simulink model "IntelligentBinPicking"  (R2024a)
settings: Solver=FixedStepAuto  StartTime=0.0  StopTime=200  FixedStep=0.05  RelTol=1e-3
PreLoadFcn:
  | initRobotModelParam;
model workspace (MAT data in the model file):
  SL_ROS_VariableLengthArrays_MaxSizes : object (value not decoded)
undefined symbols (not defined in the file): binActorRotationSequenceInfo, binActorTranslationSequenceInfo, binCenterPosition, camera_rot, cameraIntrinsics, cx_camera, cy_camera, downSampleForTrajectoryWaypoints, Enable, enumCmd, f, graspRegionTranslation, gray, homePosition, IsAccValid, IsMoving, IsPosValid, isSingleDetection, IsValid, IsVelValid, JointAcc, JointCurrent, JointPos, JointTrajectory, JointVel, maxVisionObjects, Mode, motionPlannerCmdInitValue, motionPlannerResponseInitValue, NumObjects, NumPoints, objectDetectorResponseInitValue, Objects, ObjectTypesID, pickAllOrder, PickAllOrder, PickAndPlaceModes, PickSelectedObjectID, posTargetError, predictionConfidenceScore, RequestID, Reset, RGBCameraTransform, robotCommandInitValue, robotFeedbackInitValue, Sim3dSensor, Status, TargetEETranslation, targetEnv, TaskPlannerSampleTime, Time, TooltipTransform, ur5e
libraries: sim3dlib x13, robotlib x6, robotmaniplib x4, robotcorelib x1, robotsim3dlib x1, sim3dcameralib x1
(part 2 of 2)

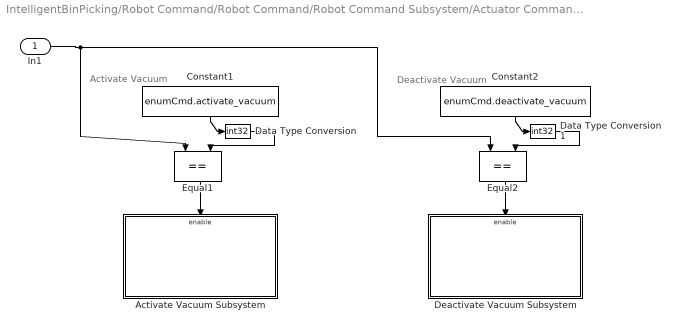
== system IntelligentBinPicking/Robot Command/Robot Command/Robot Command Subsystem/Actuator Commands/Gazebo ==
  note: Deactivate Vacuum
  note: Activate Vacuum
  In1 : Inport
  Activate Vacuum Subsystem : Subsystem
  Constant1 : Constant  Value=enumCmd.activate_vacuum
  Constant2 : Constant  Value=enumCmd.deactivate_vacuum
  Data Type Conversion : DataTypeConversion  OutDataTypeStr=int32  SaturateOnIntegerOverflow=off  RndMeth=Floor
  Data Type Conversion1 : DataTypeConversion  OutDataTypeStr=int32  SaturateOnIntegerOverflow=off  RndMeth=Floor
  Deactivate Vacuum Subsystem : Subsystem
  Equal1 : RelationalOperator  Operator===  OutDataTypeStr=boolean  RndMeth=Simplest  InputSameDT=off
  Equal2 : RelationalOperator  Operator===  OutDataTypeStr=boolean  RndMeth=Simplest  InputSameDT=off
  wires:
  Constant1/1 -> Data Type Conversion/1
  Equal2/1 -> Deactivate Vacuum Subsystem/Enable
  Constant2/1 -> Data Type Conversion1/1
  Equal1/1 -> Activate Vacuum Subsystem/Enable
  In1/1 -> Equal2/1, Equal1/1
  Data Type Conversion/1 -> Equal1/2
  Data Type Conversion1/1 -> Equal2/2

== system IntelligentBinPicking/Robot Command/Robot Command/Robot Command Subsystem/Actuator Commands/Hardware ==
  note: Activate_Deactivate Vacuum
  In1 : Inport
  Activate Vacuum Subsystem : Subsystem
  Constant1 : Constant  Value=enumCmd.activate_vacuum
  Constant2 : Constant  Value=enumCmd.deactivate_vacuum
  Data Type Conversion : DataTypeConversion  OutDataTypeStr=int32  SaturateOnIntegerOverflow=off  RndMeth=Floor
  Data Type Conversion1 : DataTypeConversion  OutDataTypeStr=int32  SaturateOnIntegerOverflow=off  RndMeth=Floor
  Equal1 : RelationalOperator  Operator===  OutDataTypeStr=boolean  RndMeth=Simplest  InputSameDT=off
  Equal2 : RelationalOperator  Operator===  OutDataTypeStr=boolean  RndMeth=Simplest  InputSameDT=off
  OR : Logic  Operator=OR  AllPortsSameDT=off  OutDataTypeStr=boolean
  wires:
  Constant1/1 -> Data Type Conversion1/1
  Equal1/1 -> OR/1
  In1/1 -> Equal1/2, Equal2/1
  Constant2/1 -> Data Type Conversion/1
  Equal2/1 -> OR/2
  OR/1 -> Activate Vacuum Subsystem/Enable
  Data Type Conversion/1 -> Equal2/2
  Data Type Conversion1/1 -> Equal1/1

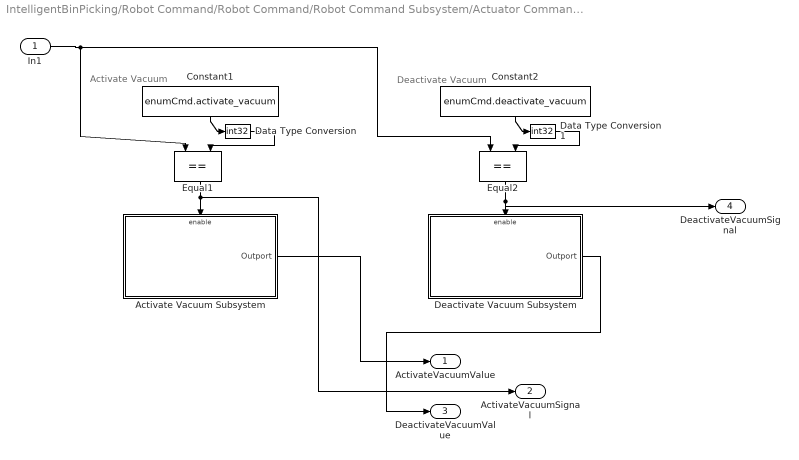
== system IntelligentBinPicking/Robot Command/Robot Command/Robot Command Subsystem/Actuator Commands/Sim3d ==
  note: Deactivate Vacuum
  note: Activate Vacuum
  In1 : Inport
  Activate Vacuum Subsystem : Subsystem
  Constant1 : Constant  Value=enumCmd.activate_vacuum
  Constant2 : Constant  Value=enumCmd.deactivate_vacuum
  Data Type Conversion : DataTypeConversion  OutDataTypeStr=int32  SaturateOnIntegerOverflow=off  RndMeth=Floor
  Data Type Conversion1 : DataTypeConversion  OutDataTypeStr=int32  SaturateOnIntegerOverflow=off  RndMeth=Floor
  Deactivate Vacuum Subsystem : Subsystem
  Equal1 : RelationalOperator  Operator===  OutDataTypeStr=boolean  RndMeth=Simplest  InputSameDT=off
  Equal2 : RelationalOperator  Operator===  OutDataTypeStr=boolean  RndMeth=Simplest  InputSameDT=off
  ActivateVacuumValue : Outport
  ActivateVacuumSignal : Outport  Port=2
  DeactivateVacuumValue : Outport  Port=3
  DeactivateVacuumSignal : Outport  Port=4
  wires:
  Constant1/1 -> Data Type Conversion/1
  Equal2/1 -> DeactivateVacuumSignal/1, Deactivate Vacuum Subsystem/Enable
  Constant2/1 -> Data Type Conversion1/1
  Equal1/1 -> ActivateVacuumSignal/1, Activate Vacuum Subsystem/Enable
  In1/1 -> Equal2/1, Equal1/1
  Data Type Conversion/1 -> Equal1/2
  Data Type Conversion1/1 -> Equal2/2
  Activate Vacuum Subsystem/1(Outport) -> ActivateVacuumValue/1
  Deactivate Vacuum Subsystem/1(Outport) -> DeactivateVacuumValue/1

== system IntelligentBinPicking/Robot Command/Robot Command/Robot Command Subsystem/Actuator Commands/Gazebo/Activate Vacuum Subsystem ==
  Enable : EnablePort
  Activate Vacuum : robotlib/Call Service  topicSource=Select from ROS network  service=/ur5/epick1/on  serviceType=std_srvs/Empty  connectionTimeout=5  keepPersistent=off  ShowErrorCodeOutput=on  legacyBusStruct=off
  Blank Message : robotlib/Blank Message  messageClass=Service Request  entityType=std_srvs/Empty  messageType=std_srvs/EmptyRequest  SampleTime=inf  legacyBusStruct=off
  wires:
  Blank Message/1 -> Activate Vacuum/1

== system IntelligentBinPicking/Robot Command/Robot Command/Robot Command Subsystem/Actuator Commands/Gazebo/Deactivate Vacuum Subsystem ==
  Enable : EnablePort
  Blank Message : robotlib/Blank Message  messageClass=Service Request  entityType=std_srvs/Empty  messageType=std_srvs/EmptyRequest  SampleTime=inf  legacyBusStruct=off
  Deactivate Vacuum : robotlib/Call Service  topicSource=Select from ROS network  service=/ur5/epick1/off  serviceType=std_srvs/Empty  connectionTimeout=5  keepPersistent=off  ShowErrorCodeOutput=on  legacyBusStruct=off
  wires:
  Blank Message/1 -> Deactivate Vacuum/1

== system IntelligentBinPicking/Robot Command/Robot Command/Robot Command Subsystem/Actuator Commands/Hardware/Activate Vacuum Subsystem ==
  Enable : EnablePort
  Activate_Deactivate Vacuum : robotlib/Call Service  topicSource=Specify your own  service=/ur_hardware_interface/hand_back_control  serviceType=std_srvs/Trigger  connectionTimeout=5  keepPersistent=off  ShowErrorCodeOutput=on  legacyBusStruct=off
  Blank Message : robotlib/Blank Message  messageClass=Service Request  entityType=std_srvs/Trigger  messageType=std_srvs/TriggerRequest  SampleTime=inf  legacyBusStruct=off
  wires:
  Blank Message/1 -> Activate_Deactivate Vacuum/1

== system IntelligentBinPicking/Robot Command/Robot Command/Robot Command Subsystem/Actuator Commands/Sim3d/Activate Vacuum Subsystem ==
  Enable : EnablePort
  Constant : Constant  OutDataTypeStr=boolean
  Outport : Outport
  wires:
  Constant/1 -> Outport/1

== system IntelligentBinPicking/Robot Command/Robot Command/Robot Command Subsystem/Actuator Commands/Sim3d/Deactivate Vacuum Subsystem ==
  Enable : EnablePort
  Constant : Constant  Value=0  OutDataTypeStr=boolean
  Outport : Outport
  wires:
  Constant/1 -> Outport/1

== matlab function IntelligentBinPicking/Robot Command/Robot Configuration  Manager/getLastPlannerWaypointConfiguration fcn ==
  data: trajectoryWaypoint input; lastPlannerWaypointConfiguration output size=[1,6]
function lastPlannerWaypointConfiguration = getLastPlannerWaypointConfiguration(trajectoryWaypoint)
lastPlannerWaypointConfiguration=zeros(1,6);
if size(trajectoryWaypoint,2) ==1
    ind=1;
else
    ind=find(all(trajectoryWaypoint == 0), 1, 'first')-1;
end
pose=trajectoryWaypoint(:,ind)';
lastPlannerWaypointConfiguration(1,1:6)=pose;

== matlab function IntelligentBinPicking/Robot Command/Robot Configuration  Manager/getGripperStatus fcn ==
  data: gripperStatus output size=[1,1]; flagG1 input; flagG2 input; graspGT input
function gripperStatus = getGripperStatus(flagG1,flagG2,graspGT)

% Persistent variable to contains state in between fcn call
persistent resultGripper;
persistent flag1GLastStatus;
persistent flag2GLastStatus;
persistent graspGTLastStatus;
if isempty (resultGripper)
    resultGripper =0;
    flag1GLastStatus= false;
    flag2GLastStatus = false;
    graspGTLastStatus =true;
end
if flagG1 || graspGT
    resultGripper= 1;
    flag1GLastStatus = flagG1;
    flag2GLastStatus = false;
    graspGTLastStatus =true;
elseif flag1GLastStatus && ~flagG2
    resultGripper=1; 
end
if flagG1 && flagG2
    resultGripper =1;
end

if ~flagG1 && ~flagG2 && ~flag2GLastStatus && ~flag1GLastStatus
    if graspGTLastStatus
        resultGripper =1;
    else
        resultGripper =0 ;
    end
end

if flagG2 
    resultGripper= 0;
    flag2GLastStatus = flagG2;
    flag1GLastStatus = false;
    graspGTLastStatus =false;
elseif flag2GLastStatus && ~flagG1
    resultGripper=0; 
end

gripperStatus = resultGripper;

== matlab function IntelligentBinPicking/Robot Command/Robot Configuration  Manager/getTrajectoryStatus fcn ==
  data: trajectoryStatus output size=[1,1]; flag1 input; flag2 input
function trajectoryStatus = getTrajectoryStatus(flag1,flag2)

% Persistent variable to contain state in between fcn call
persistent resultTrajectory;
persistent flag1LastStatus;
persistent flag2LastStatus;
if isempty (resultTrajectory)
    resultTrajectory =0;
    flag1LastStatus= false;
    flag2LastStatus = false;
end
if flag1 
    resultTrajectory= 1;
    flag1LastStatus = flag1;
    flag2LastStatus = false;
elseif flag1LastStatus && ~flag2
    resultTrajectory=1; 
end
if flag1 && flag2
    resultTrajectory =1;
end

if ~flag1 && ~flag2 && ~flag2LastStatus && ~flag1LastStatus
    resultTrajectory =0;
end

if flag2 
    resultTrajectory= 0;
    flag2LastStatus = flag2;
    flag1LastStatus = false;
elseif flag2LastStatus && ~flag1
    resultTrajectory=0; 
end

trajectoryStatus = resultTrajectory;

== matlab function IntelligentBinPicking/Object Detector/MATLAB Function ==
  data: objectDetectorResponseIn input Bus: BUS_object_detector_response; objectPose input; objectResponseOut output Bus: BUS_motion_planner_collision_object size=[maxVisionObjects 1]
function objectResponseOut = setObjectDetectedBus(objectDetectorResponseIn,objectPose)

objectResponseOut = objectDetectorResponseIn.Objects;
for i=1:size(objectPose,1)
    objectResponseOut(i).PickPos = objectPose(i, 1:3)';
    objectResponseOut(i).PickEulZYX = [objectPose(i, 4);0;0];
    objectResponseOut(i).ID = ObjectTypesID(objectPose(i, 5));
end

== matlab function IntelligentBinPicking/Robot Command/Robot Configuration  Manager/getRobotConfig fcn ==
  data: trajectoryWaypoint input; robotConfig output size=[6,1]; flag input; homePosition input; subSample input; tasks input
function robotConfig = getRobotConfig(trajectoryWaypoint,flag,homePosition,subSample,tasks)

% Persistent variable to contain state between fcn call
persistent index;
persistent lastTasksStatus;
if isempty (index)
    index=1;   
    trajectoryWaypoint= homePosition;
    lastTasksStatus = ['Place' char(repmat(' ', 1, 251))];
end
type = tasks(1).Type;
type = char(type(type~=0));
if flag 

    if ~strncmp(type,lastTasksStatus,length(type))
        index =1;
    end

    taskStatusPadded = [type char(repmat(' ', 1, 256-length(type)))];
    lastTasksStatus = taskStatusPadded(1:256);

    if strncmp(type, 'Place',5) && size(trajectoryWaypoint,2) ==1
        index =1;
    end
    
end


if ~isempty(trajectoryWaypoint)
    robotConfig = trajectoryWaypoint(1:6,index);
else
    robotConfig = homePosition;
end

if index <=size(trajectoryWaypoint,2)
    index =index + subSample;
    if index >=size(trajectoryWaypoint,2)
        index = size(trajectoryWaypoint,2);
    end
else
    index = size(trajectoryWaypoint,2);
end

== matlab function IntelligentBinPicking/Robot Command/Robot Configuration  Manager/getTargetBinActorName fcn ==
  data: u input; targetBinActorName output string; actorTranslationConfig input; actorRotationConfig input; targetBinActorOrientation output
function [targetBinActorName, targetBinActorOrientation] = getTargetBinActorName(u,actorTranslationConfig,actorRotationConfig)
translation=u(1:3,4)';

minDistance = inf; % Adjust the tolerance as needed
minIndex = 1;
for i = 1:size(actorTranslationConfig, 1)
    % distance = max(abs(givenConfigValues - bins(i, :)'));
    distance = norm(translation(1,1:2) - actorTranslationConfig(i, 1:2)*[1 0 ; 0 -1]);
    if distance < minDistance
        minDistance = distance;
        minIndex = i;
    end
end

if minIndex > 0
    out = string(sprintf('binActor%d', int8(minIndex)));
else
    out = string(sprintf('binActor%d', int8(1)));
end
targetBinActorName=out;
targetBinActorOrientation = [actorRotationConfig(minIndex,1),0,0];

== stateflow chart IntelligentBinPicking/TaskPlanner/Chart ==
  state Setup
    entry:
    ii = 1;
    obsObjectCounter = 1;
    MotionPlannerCmd = motionPlannerCmdInitValue;
    RobotCommand = robotCommandInitValue;
    pickAllObjectIndex = uint32(1);
    objectToPickIndex  = uint32(0);
    objectPickedIndices = zeros(1,maxVisionObjects);
    isVacuumOn = false;
    SimFailed = false;
  state DeactivateVacuum
    entry:
    disp('Sending Deactivate Vacuum Command');
    RobotCommand.CommandToProcess = int32(enumCmd.deactivate_vacuum);
    RobotCommand.ProcessCommand = true;
    exit:
    RobotCommand.ProcessCommand = false;
    isVacuumOn = false;
  state SendToHome
    entry:
    disp('Sending robot to home position');
    RobotCommand.CommandToProcess = int32(enumCmd.send_to_home);
    RobotCommand.ProcessCommand = true;
    exit:
    RobotCommand.ProcessCommand = false;
  state ObjectDetectorFailed
    entry:
    disp(" ");
    disp(" ");
    disp("No objects detected");
    SimFailed = true;
  state DetectObjects
    state SendObjectDetectorRequest
      en: ObjectDetectorRequest;
      disp('Object Detection in Progress');
      %du: ObjectDetectorRequest;
    state ExtractObjectToPickSingleDetection
      en:
      motionCmdWithCollisionObjects = addCollisionObjectsInfo(ObjectDetectorResponse);
      generateDroppingPoses(ObjectDetectorResponse);
      [isObjectInScene, objectToPickPos, objectToPickEul, objectToPickIndex, pickAllObjectIndex] = getObjectToPick(UserCommand, ObjectDetectorResponse, pickAllObjectIndex);
    (junction 417) -> ExtractObjectToPickSingleDetection [order 1] : [isSingleDetection == true && UserCommand.Enable == true && ObjectDetectorResponse.Status == 1 && ...
        | ObjectDetectorResponse.NumObjects >= 1]
    (junction 417) -> SendObjectDetectorRequest [order 2]
    ExtractObjectToPickSingleDetection -> SendObjectDetectorRequest [order 3]
    SendObjectDetectorRequest -> ExtractObjectToPickSingleDetection [order 2] : [UserCommand.Enable == true && ObjectDetectorResponse.Status == 1 && ...
        | ObjectDetectorResponse.NumObjects >= 1]
    ExtractObjectToPickSingleDetection -> (junction 438) [order 2] : [isObjectInScene == true]
  state StopSimulation
    entry:
    objectPickedIndices = zeros(1, maxVisionObjects);
    Stop();
  state GoToPickingPose
    state GetPickingTrajectoryFromMotionPlanner
      entry:
      % Here based on object Pos and Eul get picking pose
      pickPos = objectToPickPos + [0.0; 0.0; 0.01];  % Bring the arm to 1cm above the pick position
      pickEul = objectToPickEul;
      %Create a motion planner task bus
      MotionPlannerCmd = createMotionTask(int32(objectToPickIndex), 'Pick', uint32(300), 0.2, RobotFeedback.JointPos, pickPos, objectToPickEul);
      % Add obstacle objects
      MotionPlannerCmd.NumObstacleObjects = ObjectDetectorResponse.NumObjects - 1;
      ii= 1;
      obsObjectCounter = 1;
      for ii = 1:(ObjectDetectorResponse.NumObjects)
      if objectToPickIndex ~= ii
      MotionPlannerCmd.ObstacleObjects(obsObjectCounter) = ObjectDetectorResponse.Objects(ii);
      obsObjectCounter = obsObjectCounter + 1;
      end
      end
      % Send request to motion planner
      MotionPlannerRequest;
    state SendPickingTrajectoryToRobot
      entry:
      % Send trajectory to driver
      disp("Send traj to robot");
      RobotCommand.JointTrajectory = MotionPlannerResponse.JointTrajectory;
      RobotCommand.CommandToProcess = int32(enumCmd.precomputed_joint_trj);
      RobotCommand.ProcessCommand = true;
      posErr = Inf;
      orErr = Inf;
      success = false;
      during:
      RobotCommand.ProcessCommand = false;
      %  Check error and exit when tooltip reaches desired pose.
      T_task = eul2tform(pickEul');
      T_task(1:3,4) = pickPos;
      if targetEnv == TargetEnvs.Gazebo || targetEnv == TargetEnvs.Sim3d
      [posErr, orErr] = calcTaskSE3MaxError(T_task, RobotFeedback.TooltipTransform);
      if posErr < posTargetError
      success = true;
      end
      else
      success = ~RobotFeedback.IsMoving;
      end
      exit:
    GetPickingTrajectoryFromMotionPlanner -> (junction 14) : [MotionPlannerResponse.RequestID == MotionPlannerCmd.RequestID]
    (junction 14) -> SendPickingTrajectoryToRobot [order 1] : [MotionPlannerResponse.Status == 1 && ...
        | MotionPlannerResponse.IsPosValid == 1 && ...
        | MotionPlannerResponse.IsVelValid == 1 &&...
        |  MotionPlannerResponse.IsAccValid == 1]
  state MotionPlannerFailed
    en:
    disp('Motion Planner failed');
    SimFailed = true;
  state ActivateVacuum
    entry:
    disp('Sending Activate Vacuum Command');
    RobotCommand.CommandToProcess = int32(enumCmd.activate_vacuum);
    RobotCommand.ProcessCommand = true;
    exit:
    RobotCommand.ProcessCommand = false;
    isVacuumOn = true;
  state GoToDroppingPose
    state RequestDroppingTrajectoryFromMotionPlanner
      entry:
      droppingPose = getDroppingPose(ObjectDetectorResponse,objectToPickIndex,droppingPoses, RobotFeedback.TooltipTransform);
      % Create motion planner task bus
      MotionPlannerCmd = createMotionTask(int32(objectToPickIndex), 'Place', uint32(300), 0.2, RobotFeedback.JointPos, droppingPose(1:3), droppingPose(4:6));
      % Add obstacle objects
      MotionPlannerCmd.NumObstacleObjects = ObjectDetectorResponse.NumObjects - 1;
      ii= 1;
      obsObjectCounter = 1;
      for ii = 1:(ObjectDetectorResponse.NumObjects)
      if objectToPickIndex ~= ii
      MotionPlannerCmd.ObstacleObjects(obsObjectCounter) = ObjectDetectorResponse.Objects(ii);
      obsObjectCounter = obsObjectCounter + 1;
      end
      end
      % Send request to motion planner
      MotionPlannerRequest;
    state SendDroppingTrajectoryToRobot
      entry:
      % Send trajectory to driver
      RobotCommand.JointTrajectory = MotionPlannerResponse.JointTrajectory;
      RobotCommand.CommandToProcess = int32(enumCmd.precomputed_joint_trj);
      RobotCommand.ProcessCommand = true;
      posErr = Inf;
      orErr = Inf;
      success = false;
      during:
      RobotCommand.ProcessCommand = false;
      %  Check error and exit when tooltip reaches desired pose.
      T_task = eul2tform(droppingPose(4:6)');
      T_task(1:3,4) = droppingPose(1:3);
      if targetEnv == TargetEnvs.Gazebo || targetEnv == TargetEnvs.Sim3d
      [posErr, orErr] = calcTaskSE3MaxError(T_task, RobotFeedback.TooltipTransform);
      if posErr < posTargetError
      success = true;
      end
      else
      success = ~RobotFeedback.IsMoving;
      end
      exit:
    RequestDroppingTrajectoryFromMotionPlanner -> (junction 128) : [MotionPlannerResponse.RequestID == MotionPlannerCmd.RequestID]
    (junction 128) -> SendDroppingTrajectoryToRobot [order 1] : [MotionPlannerResponse.Status == 1 && ...
        | MotionPlannerResponse.IsPosValid == 1 && ...
        | MotionPlannerResponse.IsVelValid == 1 && ...
        | MotionPlannerResponse.IsAccValid == 1]
  state Stop [function]
  SendPickingTrajectoryToRobot -> ActivateVacuum : [success == true]
  SendToHome -> (junction 417) [order 2]
  ActivateVacuum -> RequestDroppingTrajectoryFromMotionPlanner : {pause(0.5)}
  ExtractObjectToPickSingleDetection -> StopSimulation [order 1] : [objectToPickIndex == uint32(-1)]
      | {disp('No more objects to pick. Stopping simulation')}
  (junction 438) -> GetPickingTrajectoryFromMotionPlanner : {pause(1)}
  (default) -> Setup
  Setup -> (junction 498) : [UserCommand.Enable == true && RobotFeedback.IsValid]
  (junction 498) -> (junction 500) [order 2] : [nnz(objectPickedIndices) == 0]
  (junction 498) -> DeactivateVacuum [order 1] : [nnz(objectPickedIndices) > 0]
  (junction 500) -> SendToHome
  (junction 253) -> (junction 519)
  (junction 519) -> DeactivateVacuum [order 1] : [isVacuumOn == true]
  (junction 535) -> (junction 253)
  (junction 519) -> SendToHome [order 2]
  DeactivateVacuum -> SendToHome : {pause(1)}
  SendToHome -> (junction 532) [order 1] : [SimFailed == true]
  (junction 532) -> StopSimulation : {disp('Stopping simulation')}
  ObjectDetectorFailed -> (junction 535)
  (junction 527) -> (junction 535)
  SendDroppingTrajectoryToRobot -> (junction 256) : [success == true]
  MotionPlannerFailed -> (junction 527)
  (junction 485) -> (junction 527)
  SendObjectDetectorRequest -> ObjectDetectorFailed [order 1] : [ObjectDetectorResponse.Status == -1]
  (junction 256) -> (junction 485)
  (junction 128) -> MotionPlannerFailed [order 2]
  (junction 14) -> MotionPlannerFailed [order 2]
  data: requestIDIn function_input; typeIn function_input; maxIterationsIn function_input; sampleTimeIn function_input; q0In function_input; targetPosIn function_input; targetEulIn function_input; motionPlannerCmdOut function_output; T_aIn function_input double size=[4 4]; T_bIn function_input double size=[4 4]; posErrOut function_output double size=1; orErrOut function_output double size=1; objectDetectorResponse function_input; droppingPoseOut function_output double size=[6 1]; ObjectDetectorResponseIn function_input Bus: BUS_object_detector_response size=1; objectToPickIdx function_input; droppingPosesIn function_input size=[6, maxVisionObjects]; unused function_input; detectorResponse function_input; motionCmd function_output; userCommandIn function_input Bus: BUS_user_command size=1; objectDetectorResponseIn function_input Bus: BUS_object_detector_response size=1; isObjectInSceneOut function_output; objectToPickPosOut function_output double size=[3 1]; objectToPickEulOut function_output double size=[3 1]; objectToPickIndexOut function_output uint32 size=1; pickAllObjectIndexOut function_output uint32 size=1; pickAllObjectIndexIn function_input uint32 size=1; RobotCommand output Bus: BUS_robot_command size=1; UserCommand input Bus: BUS_user_command size=1; ObjectDetectorResponse input Bus: BUS_object_detector_response size=1; MotionPlannerResponse input Bus: BUS_motion_planner_response size=1; MotionPlannerCmd output Bus: BUS_motion_planner_cmd size=1; isObjectInScene local boolean size=1 =false; objectToPickEul local; objectToPickPos local; ii local uint32 size=1; obsObjectCounter local uint32 size=1; RobotFeedback input Bus: BUS_robot_feedback size=1; T_task local double size=[4, 4]; orErr local double size=1; posErr local double size=1; posTargetError parameter double size=1; droppingPoses local double size=[6, maxVisionObjects] =zeros(6, maxVisionObjects); pickEul local double size=[3 1]; pickPos local double size=[3 1]; pickAllObjectIndex local uint32 size=1; objectToPickIndex local uint32 size=1; droppingPose local double size=[6 1]; robotCommandInitValue parameter size=1; isSingleDetection parameter; binCenterPosition parameter; objectPickedIndices local double size=[1 maxVisionObjects] =zeros(1, maxVisionObjects); targetEnv parameter; motionCmdWithCollisionObjects local Bus: BUS_motion_planner_cmd size=1; success local; maxVisionObjects parameter double size=1; isVacuumOn local boolean size=1 =false; SimFailed local boolean size=1 =false; motionPlannerCmdInitValue parameter size=1
  events: MotionPlannerRequest output FUNCTION_CALL_EVENT; ObjectDetectorRequest output FUNCTION_CALL_EVENT
  function motionPlannerCmdOut = createMotionTask(requestIDIn, typeIn, maxIterationsIn, sampleTimeIn, q0In, targetPosIn, targetEulIn):
    | function motionPlannerCmdOut = createMotionTask(requestIDIn, typeIn, maxIterationsIn, sampleTimeIn, q0In, targetPosIn, targetEulIn)
    | 
    | % In this one I didn't expose the max velocity because the planner doesn't
    | % consider the acceleration limits directly. We use a conservative Lin and
    | % Ang limits to control acceleration.
    | 
    | % q0In = [q0In; 0; 0; 0; 0; 0; 0;];
    | 
    | % Initialize bus
    | motionPlannerCmdOut = motionCmdWithCollisionObjects;
    | 
    | % Configure motion planner tasks
    | motionPlannerCmdOut.RequestID = requestIDIn;
    | motionPlannerCmdOut.NumTasks = uint32(4);
    | motionPlannerCmdOut.MaxIterations = maxIterationsIn;
    | motionPlannerCmdOut.SampleTime = sampleTimeIn;
    | motionPlannerCmdOut.InitialPositions = q0In;
    | % Task 1: End effector pose
    | motionPlannerCmdOut.Tasks(1).Name(1:length(uint8('TooltipTaskSE3'))) = uint8('TooltipTaskSE3');
    | motionPlannerCmdOut.Tasks(1).Type(1:length(typeIn))  = uint8(typeIn);
    | motionPlannerCmdOut.Tasks(1).FrameName(1:length(uint8('Bellow')))  = uint8('Bellow');
    | motionPlannerCmdOut.Tasks(1).p = targetPosIn;
    | motionPlannerCmdOut.Tasks(1).eulZYX = targetEulIn;
    | motionPlannerCmdOut.Tasks(1).MaxLinVel = 0.10;  % 0.072 0.1 0.15
    | motionPlannerCmdOut.Tasks(1).MaxAngVel = 0.4;    % 0.4
    | motionPlannerCmdOut.Tasks(1).Weight = 1.0;
    | motionPlannerCmdOut.Tasks(1).MaxLinError = 0.01;        % 0.01
    | motionPlannerCmdOut.Tasks(1).MaxAngError = deg2rad(2);  % 2
  function [posErrOut,orErrOut] = calcTaskSE3MaxError(T_aIn, T_bIn):
    | function [posErrOut,orErrOut] = calcTaskSE3MaxError(T_aIn, T_bIn)
    |  
    | % Position error is max of coordinate
    | posErrOut = max(abs(T_aIn(1:3,4) - T_bIn(1:3,4)));
    | 
    | % Orientation error with quaternions. Also using max for error
    | q_a = tform2quat(T_aIn);
    | q_b = tform2quat(T_bIn);
    | 
    | % skew
    | S_a = [      0, -q_a(4),  q_a(3); 
    |         q_a(4),       0, -q_a(2); 
    |        -q_a(3),  q_a(2),       0];
    |     
    | or_error = q_b(1)*q_a(2:4)'-q_a(1)*q_b(2:4)'- S_a*q_b(2:4)';    % q = [w x y z]
    | 
    | orErrOut = max(abs(or_error));
  function generateDroppingPoses(objectDetectorResponse):
    | function generateDroppingPoses(objectDetectorResponse)
    |  
    | %% Define dropping poses
    | 
    | 
    | %For single detection workflow, the dropping poses will get defined once
    | %and then used in the getDroppingPoses method.
    | 
    | %For multiple detections, ensure that the dropping poses get generated only
    | %once. Check the presence of non-zero value in objectPickedIndices to
    | %detect subsequent detections.
    | 
    | %In this implementation, the user defined drop POSITION doesn't change based
    | %on the pose of the object before picking. However, the orientation of the object
    | %may change during the course of picking other objects and that is taken
    | %into account in the getDroppingPose method.
    | 
    | %Generate dropping pose only once
    | if isempty(find(objectPickedIndices,1))
    |     numOfParts = objectDetectorResponse.NumObjects;
    |     droppingPoses = zeros(6, maxVisionObjects);
    |     for i=1:numOfParts
    |         if i>numOfParts-1
    |             droppingPoses(:, i) = [0.01 0.59 -0.018 0 pi 0]';
    |         else
    |             droppingPoses(:, i) = [0.01+(double(i)-1)*0.07 0.75 -0.018 0 pi 0]';
    |         end
    |     end
    | end
  function droppingPoseOut = getDroppingPose(ObjectDetectorResponseIn,objectToPickIdx,droppingPosesIn,~):
    | function droppingPoseOut = getDroppingPose(ObjectDetectorResponseIn,objectToPickIdx,droppingPosesIn,~)
    | 
    | % Use the number of objects already picked to determine the dropping pose
    | % for the current object
    | droppingPoseOut = droppingPosesIn(:,objectToPickIdx);
    | 
    | objClass = string(ObjectTypesID(ObjectDetectorResponseIn.Objects(objectToPickIdx).ID));
    | %droppingPoseOut = zeros(1,6);
    |     if  objClass == 'I'
    |         droppingPoseOut(1:3) = [0.1 0.6 0.07];
    |     elseif objClass == 'X'
    |         droppingPoseOut(1:3) = [0.4 0.6 0.07];
    |     elseif objClass == 'T'
    |         droppingPoseOut(1:3) = [0.4 -0.6 0.07];
    |     else
    |         droppingPoseOut(1:3) = [0.1 -0.6 0.07];
    |     end
    | %Take into account the orientation of the object in the bin
    | droppingPoseOut(4) = 0;
  function motionCmd = addCollisionObjectsInfo(detectorResponse):
    | function motionCmd = addCollisionObjectsInfo(detectorResponse)
    | 
    | motionCmd = motionPlannerCmdInitValue;
    | 
    | numObjectsToPick = detectorResponse.NumObjects;
    | motionCmd.NumObstacleObjects = numObjectsToPick;
    | 
    | for ii = 1:numObjectsToPick
    |    motionCmd.ObstacleObjects(ii) = detectorResponse.Objects(ii);
    | end
    | 
    | 
    | end
  function [isObjectInSceneOut, objectToPickPosOut, objectToPickEulOut, objectToPickIndexOut, pickAllObjectIndexOut]=  getObjectToPick(userCommandIn,objectDetectorResponseIn, pickAllObjectIndexIn):
    | function [isObjectInSceneOut, objectToPickPosOut, objectToPickEulOut, objectToPickIndexOut, pickAllObjectIndexOut]=  getObjectToPick(userCommandIn,objectDetectorResponseIn, pickAllObjectIndexIn)
    |  
    | isObjectInSceneOut = false;
    | objectToPickPosOut = zeros(3,1);
    | objectToPickEulOut = zeros(3,1);
    | objectToPickIndexOut = uint32(0);
    | pickAllObjectIndexOut = pickAllObjectIndexIn;
    | 
    | %If a single detection is being done, then we need to keep track of which
    | %objects were picked, objectPickedIndices. On the othe rhand, when doing a
    | %detection after each pick and place operation, we just need to pick up the
    | %object closest to the center of the bin.
    | if isSingleDetection
    |     % List of parts poses that are still in the bin
    |     partsToPickGT = zeros(objectDetectorResponseIn.NumObjects - nnz(objectPickedIndices), 6);
    |     if ~isempty(partsToPickGT)
    |         partsToPickGTIdx = 1;
    |         partsToPickDetectedIdx = zeros(1,10);
    |         for ii = 1:objectDetectorResponseIn.NumObjects
    |             %If the part has been picked, don't use its pose
    |             if ~any(objectPickedIndices == ii)
    |                 partsToPickGT(partsToPickGTIdx, 1:3) = objectDetectorResponseIn.Objects(ii).PickPos;
    |                 partsToPickGT(partsToPickGTIdx, 4) = objectDetectorResponseIn.Objects(ii).PickEulZYX(1);
    |                 partsToPickDetectedIdx(partsToPickGTIdx) = ii;
    |                 partsToPickGTIdx = partsToPickGTIdx + 1;
    |             end
    |         end
    | 
    |         [refPose,partIDToPick] = exampleHelperSelectPartForMEXPlanner(partsToPickGT,binCenterPosition);
    |         
    |         if ~isempty(refPose)
    |             isObjectInSceneOut = true;
    |             objectToPickPosOut = refPose';
    |             objectToPickIndexOut = uint32(partsToPickDetectedIdx(partIDToPick));
    |             objectToPickEulOut = [ deg2rad(objectDetectorResponseIn.Objects(objectToPickIndexOut).PickEulZYX(1)) pi 0]';
    |             if pickAllObjectIndexIn < length(userCommandIn.PickAllOrder)
    |                 pickAllObjectIndexOut = pickAllObjectIndexIn + 1;
    |             else
    |                 pickAllObjectIndexOut = uint32(1);
    |             end
    | 
    |             if size(partsToPickGT, 1) == objectDetectorResponseIn.NumObjects
    |                 objectPickedIndices(1) = objectToPickIndexOut;
    |             else
    |                 objectPickedIndices(find(objectPickedIndices, 1, 'Last') + 1) = objectToPickIndexOut;
    |             end
    |         end
    |     else
    |         objectToPickIndexOut = uint32(-1);
    |     end
    | 
    | else
    |     partsToPickGT = zeros(objectDetectorResponseIn.NumObjects, 6);
    |     if ~isempty(partsToPickGT)
    |         for ii = 1:objectDetectorResponseIn.NumObjects
    |             partsToPickGT(ii, 1:3) = objectDetectorResponseIn.Objects(ii).PickPos;
    |             partsToPickGT(ii, 4) = objectDetectorResponseIn.Objects(ii).PickEulZYX(1);
    |         end
    | 
    |         [refPose,partIDToPick] = exampleHelperSelectPartForMEXPlanner(partsToPickGT,binCenterPosition);
    | 
    |         if ~isempty(refPose)
    |             isObjectInSceneOut = true;
    |             objectToPickPosOut = refPose';
    |             objectToPickEulOut = [0 pi 0]';
    |             objectToPickIndexOut = uint32(partIDToPick);
    |             if pickAllObjectIndexIn < length(userCommandIn.PickAllOrder)
    |                 pickAllObjectIndexOut = pickAllObjectIndexIn + 1;
    |             else
    |                 pickAllObjectIndexOut = uint32(1);
    |             end
    | 
    |             if isempty(find(objectPickedIndices,1))
    |                 objectPickedIndices(1) = partIDToPick;
    |             else
    |                 objectPickedIndices(find(objectPickedIndices, 1, 'Last') + 1) = partIDToPick;
    |             end
    |         end
    |     else
    |         objectToPickIndexOut = uint32(-1);
    |     end
    | end
